simulink model "SSModel"  (R2016b)
settings: Solver=VariableStepAuto  StartTime=0.0  StopTime=3.5  RelTol=1e-3
values from neighbouring files (symbols this model uses):
  A = [ 0 1 0 ... (first row only)    [CubeEdge.m]    (also in accelscript.m = (r*(((theta-theta1)/Ts) - ((theta1-theta2)/Ts))/Ts) + g*thet; testscript.m)
  B = [ 0 ... (first row only)    [CubeEdge.m]    (also in accelscript.m = simplify( solve(A, theta)); testscript.m)
  C = eye(3)    [CubeEdge.m]    (also in testscript.m)
  D = zeros(3,1)    [CubeEdge.m]    (also in testscript.m)
  K = place(A,B,P)    [CubeEdge.m]    (also in testscript.m; tfscript.m = [ 0 0 0 0 0 1]*inv(M)*Phi)
settings Model: Creator=Will  LastModifiedBy=Will
settings DataIOCC: Refine=5

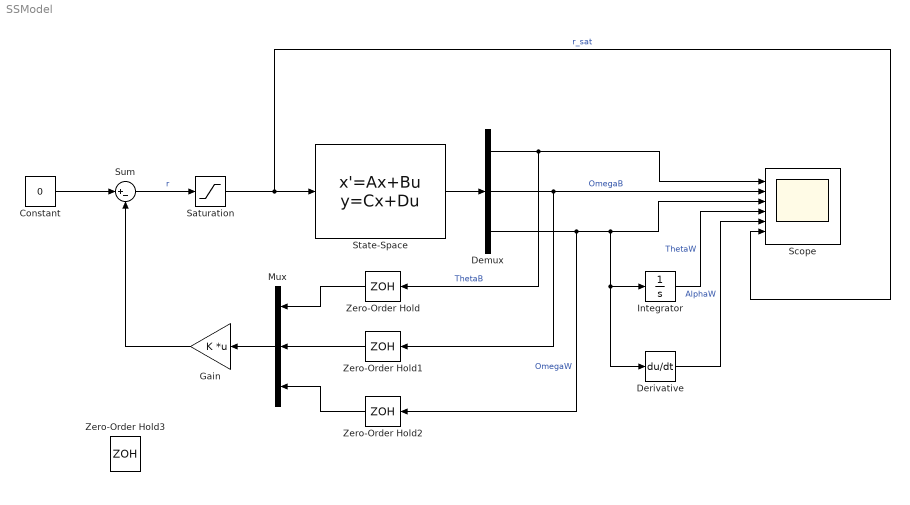
== system SSModel ==
  Constant : Constant  Value=0
  Demux : Demux  Outputs=3
  Derivative : Derivative
  Gain : Gain  Gain=K  Multiplication=Matrix(K*u)
  Integrator : Integrator
  Mux : Mux  Inputs=3
  Saturation : Saturate  UpperLimit=6  LowerLimit=-6
  Scope : Scope  NumInputPorts=6
  State-Space : StateSpace  A=A  B=B  C=C  D=D  X0=[.1 0 0]  ContinuousStateAttributes={'ThetaB', 'OmegaB', 'OmegaW'}
  Sum : Sum  Inputs=|+-
  Zero-Order Hold : ZeroOrderHold  SampleTime=1/100
  Zero-Order Hold1 : ZeroOrderHold  SampleTime=1/100
  Zero-Order Hold2 : ZeroOrderHold  SampleTime=1/6500
  Zero-Order Hold3 : ZeroOrderHold  SampleTime=1/6500
  wires:
  Demux/1 -> Zero-Order Hold/1, Scope/1  "ThetaB"
  Demux/2 -> Zero-Order Hold1/1, Scope/2  "OmegaB"
  Demux/3 -> Zero-Order Hold2/1, Derivative/1, Integrator/1, Scope/3  "OmegaW"
  Sum/1 -> Saturation/1  "r"
  Constant/1 -> Sum/1
  State-Space/1 -> Demux/1
  Integrator/1 -> Scope/4  "ThetaW"
  Derivative/1 -> Scope/5  "AlphaW"
  Saturation/1 -> Scope/6, State-Space/1  "r_sat"
  Gain/1 -> Sum/2
  Mux/1 -> Gain/1
  Zero-Order Hold/1 -> Mux/1
  Zero-Order Hold1/1 -> Mux/2
  Zero-Order Hold2/1 -> Mux/3
